simulink model "usrp_1t3r_positioning"  (R2017a)
settings: Solver=VariableStepAuto  StartTime=0.0  StopTime=inf  RelTol=1e-3
undefined symbols (not defined in the file): get
libraries: dspsnks4 x5, commsdrhw_v2 x1, dspxfrm3 x1, dspstat3 x1, dspmtrx3 x1, dspsigops x1
settings Model: SimulationMode=accelerator  Creator=Sky  LastModifiedBy=Sky

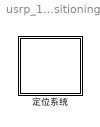
== system usrp_1t3r_positioning ==
  定位系统 : Subsystem  mask{decimInterp=100, fTr=400, nPul=3, tPul=0.1e-3, nCyclePF=5, trEdge=0, antBits=logical([0 0;1 0;0 1])}
      mask prompts: decimInterp "Decimation Factor"; fTr "triger frequency"; nPul "pulse number"; tPul "pulse time"; nCyclePF "cycles per frame (average time)"; trEdge "triger Edge"; antBits "antenna bits"
      mask init:
      | global nRx lF fS lRamp
      | nRx=size(antBits,1);
      | lF=100e6/decimInterp/fTr*nRx*nCyclePF;
      | fS=100e6/decimInterp;
      | lRamp=fS/fTr;%length ramp
      mask TypeOptions decimInterp: USRP/decimInterp
      mask TypeOptions fTr: 定位模块/fTr
      mask TypeOptions nPul: 定位模块/nPul
      mask TypeOptions tPul: 定位模块/tPul
      mask TypeOptions trEdge: 定位模块/trEdge
      mask TypeOptions antBits: 定位模块/antBits
      mask Display: disp('定位系统');

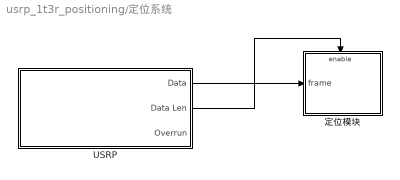
== system usrp_1t3r_positioning/定位系统 ==
  USRP : Subsystem  mask{decimInterp=decimInterp, lF=lF}
      mask prompts: decimInterp "Decimation Factor"; lF "frameLength"
      mask TypeOptions decimInterp: SDRu Receiver/decimInterp
      mask TypeOptions lF: SDRu Receiver/frameLength
      mask Display: disp('USRP');
  定位模块 : Subsystem  mask{fTr=fTr, nPul=nPul, tPul=tPul, trThres=-0.2169682, trEdge=trEdge, antBits=antBits}
      mask prompts: fTr "triger frequency"; nPul "pulse number"; tPul "pulse time"; trThres "triger Threshold"; trEdge "triger Edge"; antBits "antenna bits"
      mask Display: disp('定位模块');
  wires:
  USRP/1(Data) -> 定位模块/1(frame)
  USRP/2(Data Len) -> 定位模块/Enable

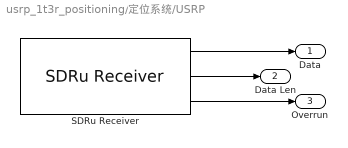
== system usrp_1t3r_positioning/定位系统/USRP ==
  SDRu Receiver : commsdrhw_v2/SDRu Receiver  SourceLibraryInfo="This block requires <a href=\"http://www.mathworks.com/hardware-support/usrp.html\">Communications System Toolbox Support Package for USRP Radio</a>"  rxtx=rx  platform=N200/N210/USRP2  USRP2_IP='192.168.10.6'  USRP_IP_X300='192.168.10.2'  USRP_IP_X310='192.168.10.2'  USRP_serialNumB200=''  USRP_serialNumB210=''  ChannelMapping=1  centerFrequency=0  centerFrequencySrc=Dialog  loOffset=0  loOffsetSrc=Dialog  PPSSource=Internal  clockSource=Internal  masterClkRateB200=32e6  masterClkRateB210=32e6  masterClkRateX300=200e6  masterClkRateX310=200e6  masterClkRateParam=100e6  gain=0  gainSrc=Dialog  decimInterpSrc=Dialog  decimInterp=decimInterp  TransportDataType=int16  USRP2_IP_NUM=[49 57 50 46 49 54 56 46 49 48 46 54]  frameLength=lF  outputDatatype=single  overrunUnderrunPort=on  sampleTime=decimInterp/100e6  HOST_DATA_PORT=0  HOST_CONTROL_PORT=0  USRP2_DATA_PORT=0  USRP2_CONTROL_PORT=0  bufferMode=Continuous streaming  EnableBurstMode=off  NumFramesInBurst=10000  USRP_ID='192.168.10.6'
      settings: SourceProductName=Communications System Toolbox Support Package for USRP(R) Radio  SourceProductBaseCode=USRP
  Data : Outport
  Data Len : Outport  Port=2
  Overrun : Outport  Port=3
  wires:
  SDRu Receiver/2 -> Data Len/1
  SDRu Receiver/3 -> Overrun/1
  SDRu Receiver/1 -> Data/1

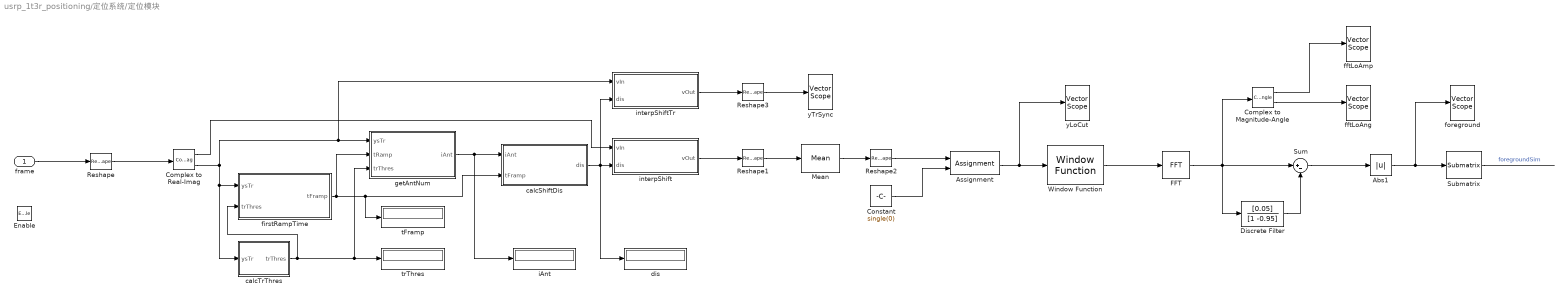
== system usrp_1t3r_positioning/定位系统/定位模块 ==
  frame : Inport
  Enable : EnablePort
  Abs1 : Abs
  Assignment : Assignment  NumberOfDimensions=2  DiagnosticForDimensions=Warning  IndexOptions=Index vector (dialog),Assign all  Indices=[1:ceil(1.5e-5*fS),lRamp-ceil(1.5e-5*fS):lRamp],1  OutputSizes=1,1
  Complex to Magnitude-Angle : ComplexToMagnitudeAngle
  Complex to Real-Imag : ComplexToRealImag
  Constant : Constant  Value=single(0)
  Discrete Filter : DiscreteFilter  Numerator=[0.05]  Denominator=[1 -0.95]
  FFT : dspxfrm3/FFT  FFTImplementation=Auto  CompMethod=Table lookup  TableOpt=NEW  TableOptActive=Speed  BitRevOrder=off  Normalize=off  InheritFFTLength=on  FFTLength=1024*16  WrapInput=on  roundingMode=Floor  overflowMode=off  firstCoeffDataTypeStr=Inherit: Same word length as input  firstCoeffLastDataTypeStr=Inherit: Same word length as input  outputMin=[]  outputMax=[]
  Mean : dspstat3/Mean  run=off  reset_popup=None  InputProcessing=Columns as channels (frame based)  directionMode=Each row  dimension=1  roiEnable=off  roiType=Rectangles  roiPortion=Entire ROI  roiOutput=Individual statistics for each ROI  roiFlag=off  outputDataTypeStr=Inherit: Same as accumulator  outputLastDataTypeStr=Inherit: Same as accumulator  outputMin=[]  outputMax=[]  roundingMode=Floor  overflowMode=off
  Reshape : Reshape  OutputDimensionality=Row vector (2-D)
  Reshape1 : Reshape  OutputDimensionality=Customize  OutputDimensions=[lRamp*nRx,nCyclePF]
  Reshape2 : Reshape  OutputDimensionality=Customize  OutputDimensions=[lRamp,nRx]
  Reshape3 : Reshape  OutputDimensionality=Column vector (2-D)
  Submatrix : dspmtrx3/Submatrix  RowSpan=Range of rows  RowStartMode=First  RowStartIndex=1  RowEndMode=Offset from middle  RowEndIndex=-1  ColSpan=All columns  ColStartMode=First  ColStartIndex=1  ColEndMode=Last  ColEndIndex=1
  Sum : Sum  Inputs=|+-
  Window Function : dspsigops/Window Function  winmode=Apply window to input  wintype=Hanning  sampmode=Continuous  samptime=1  N=64  Rs=50  beta=10  winsamp=Symmetric  UserWindow=hamming  OptParams=off  UserParams={'symmetric'}  dataType=double  isSigned=on  wordLen=16  udDataType=sfix(16)  fracBitsMode=Best precision  numFracBits=15  roundingMode=Floor  overflowMode=off  numSidelobes=4  sidelobeLevel=-30
      settings: SourceProductName=DSP System Toolbox  SourceProductBaseCode=DS
  calcShiftDis : MATLAB Function  TreatAsAtomicUnit=on
  calcTrThres : MATLAB Function  TreatAsAtomicUnit=on
  dis : Display
  fftLoAmp : dspsnks4/Vector Scope  ScopeProperties=on  Domain=Frequency  HorizSpan=1  DisplayProperties=off  AxisGrid=on  Memory=off  FrameNumber=on  AxisLegend=on  AxisZoom=off  OpenScopeAtSimStart=on  OpenScopeImmediately=off  FigPos=get(0,'defaultfigureposition')  AxisProperties=off  XUnits=Hertz  XRange=[0...Fs/2]  InheritXIncr=off  XIncr=1/fS  XLabel=Time  XLimit=Auto  XMin=0  XMax=1  XStart=0  YUnits=Magnitude  YLabel=Amplitude  LineProperties=off  LineDisables=on|on|on  LineColors=[1 0 0]|[0 1 0]|[0 0 1]  XAxisParamsVer=6.9
      settings: SourceProductName=DSP System Toolbox  SourceProductBaseCode=DS  YMin=0  YMax=50
  fftLoAng : dspsnks4/Vector Scope  ScopeProperties=on  Domain=Frequency  HorizSpan=1  DisplayProperties=off  AxisGrid=on  Memory=off  FrameNumber=on  AxisLegend=on  AxisZoom=off  OpenScopeAtSimStart=on  OpenScopeImmediately=off  FigPos=get(0,'defaultfigureposition')  AxisProperties=off  XUnits=Hertz  XRange=[0...Fs/2]  InheritXIncr=off  XIncr=1/fS  XLabel=Time  XLimit=Auto  XMin=0  XMax=1  XStart=0  YUnits=Magnitude  YLabel=Amplitude  LineProperties=off  LineDisables=on|on|on  LineColors=[1 0 0]|[0 1 0]|[0 0 1]  XAxisParamsVer=6.9
      settings: SourceProductName=DSP System Toolbox  SourceProductBaseCode=DS  YMin=-4  YMax=4
  firstRampTime : MATLAB Function  TreatAsAtomicUnit=on
  foreground : dspsnks4/Vector Scope  ScopeProperties=on  Domain=Frequency  HorizSpan=1  DisplayProperties=off  AxisGrid=on  Memory=off  FrameNumber=on  AxisLegend=on  AxisZoom=off  OpenScopeAtSimStart=on  OpenScopeImmediately=off  FigPos=get(0,'defaultfigureposition')  AxisProperties=off  XUnits=Hertz  XRange=[0...Fs/2]  InheritXIncr=off  XIncr=1/fS  XLabel=Time  XLimit=Auto  XMin=0  XMax=1  XStart=0  YUnits=Magnitude  YLabel=Amplitude  LineProperties=off  LineDisables=on|on|on  LineColors=[1 0 0]|[0 1 0]|[0 0 1]  XAxisParamsVer=6.9
      settings: SourceProductName=DSP System Toolbox  SourceProductBaseCode=DS  YMin=0  YMax=0.2
  getAntNum : MATLAB Function  TreatAsAtomicUnit=on
  iAnt : Display
  interpShift : MATLAB Function  TreatAsAtomicUnit=on
  interpShiftTr : MATLAB Function  TreatAsAtomicUnit=on
  tFramp : Display
  trThres : Display
  yLoCut : dspsnks4/Vector Scope  ScopeProperties=on  Domain=Time  HorizSpan=1  DisplayProperties=off  AxisGrid=on  Memory=off  FrameNumber=on  AxisLegend=off  AxisZoom=off  OpenScopeAtSimStart=on  OpenScopeImmediately=off  FigPos=get(0,'defaultfigureposition')  AxisProperties=off  XUnits=Hertz  XRange=[0...Fs/2]  InheritXIncr=on  XIncr=1  XLabel=Time  XLimit=Auto  XMin=0  XMax=1  XStart=0  YUnits=dB  YLabel=Amplitude  LineProperties=off  LineColors=[1 0 0]|[0 1 0]|[0 0 1]  XAxisParamsVer=6.9
      settings: SourceProductName=DSP System Toolbox  SourceProductBaseCode=DS  YMin=-0.5  YMax=0.5
  yTrSync : dspsnks4/Vector Scope  ScopeProperties=on  Domain=Time  HorizSpan=1  DisplayProperties=off  AxisGrid=on  Memory=off  FrameNumber=on  AxisLegend=off  AxisZoom=off  OpenScopeAtSimStart=on  OpenScopeImmediately=off  FigPos=get(0,'defaultfigureposition')  AxisProperties=off  XUnits=Hertz  XRange=[0...Fs/2]  InheritXIncr=on  XIncr=1  XLabel=Time  XLimit=Auto  XMin=0  XMax=1  XStart=0  YUnits=dB  YLabel=Amplitude  LineProperties=off  LineColors=[1 0 0]|[0 1 0]|[0 0 1]  XAxisParamsVer=6.9
      settings: SourceProductName=DSP System Toolbox  SourceProductBaseCode=DS  YMin=-0.6  YMax=0.2
  wires:
  firstRampTime/1(tFramp) -> tFramp/1, calcShiftDis/2(tFramp), getAntNum/2(tRamp)
  frame/1 -> Reshape/1
  Reshape/1 -> Complex to Real-Imag/1
  getAntNum/1(iAnt) -> iAnt/1, calcShiftDis/1(iAnt)
  Complex to Real-Imag/2 -> calcTrThres/1(ysTr), firstRampTime/1(ysTr), interpShiftTr/1(vIn), getAntNum/1(ysTr)
  calcShiftDis/1(dis) -> dis/1, interpShift/2(dis), interpShiftTr/2(dis)
  interpShift/1(vOut) -> Reshape1/1
  Complex to Real-Imag/1 -> interpShift/1(vIn)
  calcTrThres/1(trThres) -> trThres/1, getAntNum/3(trThres), firstRampTime/2(trThres)
  Reshape1/1 -> Mean/1
  Mean/1 -> Reshape2/1
  Discrete Filter/1 -> Sum/2
  FFT/1 -> Complex to Magnitude-Angle/1, Discrete Filter/1, Sum/1
  Sum/1 -> Abs1/1
  Abs1/1 -> Submatrix/1, foreground/1
  Complex to Magnitude-Angle/2 -> fftLoAng/1
  Reshape2/1 -> Assignment/1
  Constant/1 -> Assignment/2
  Submatrix/1 -> ?  "foregroundSim"
  Assignment/1 -> yLoCut/1, Window Function/1
  Complex to Magnitude-Angle/1 -> fftLoAmp/1
  interpShiftTr/1(vOut) -> Reshape3/1
  Reshape3/1 -> yTrSync/1
  Window Function/1 -> FFT/1

== matlab function usrp_1t3r_positioning/定位系统/定位模块/getAntNum ==
  data: ysTr input; tRamp input; iAnt output; fS parameter; tPul parameter; antBits parameter; trThres input
%% 判断触发时间对应同步信号的天线编号
% iAnt: 天线编号
% ysTr: 一帧triger信号
% tRamp: 斜坡开始时间，以第一个采样点为参考时间0
% fS: 采样率
% tPul: 脉冲/比特宽度
% trThres: 触发电平
% antBits: 天线编号
function iAnt=getAntNum(ysTr, tRamp, fS, tPul, antBits, trThres)
if isnan(tRamp)
    iAnt=nan;
    return
end
%% 准备参数
lPul=fS*tPul;%length pulse

%% 抽取天线编号的比特电平
iBit1=ceil((tRamp+1.5*tPul)*fS)+1;
isBits=linspace(iBit1,iBit1+lPul*(size(antBits,2)-1),size(antBits,2));

ysBits=ysTr(isBits);
isAnt=find(all(~xor(antBits,repmat((ysBits>trThres),size(antBits,1),1)),2),1);
if isempty(isAnt)
    iAnt=nan;
    return
end
iAnt=isAnt(1);%为simulink推理iAnt大小提供帮助

end

== matlab function usrp_1t3r_positioning/定位系统/定位模块/firstRampTime ==
  data: ysTr input; tFramp output; fS parameter; fTr parameter; tPul parameter; nPul parameter; trEdge parameter; trThres input
%% 同步斜坡信号起始时间函数，返回所有斜坡信号起始时间点
% tFramp: 第一个斜坡开始时间，精确到采样时间之下，以第一个采样点为参考时间0
% ysTr: 一帧triger信号
% fS: 采样率
% fTr: 触发信号频率
% tPul: 脉冲/比特宽度
% nPul: 脉冲/比特总数
% trEdge: 触发沿：1上升沿 0下降沿
% trThres: 触发电平
function tFramp=firstRampTime(ysTr, fS, fTr, tPul, nPul, trEdge, trThres)
%% 准备参数
lRamp=fS/fTr;%length ramp
lPul=fS*tPul;%length pulse

if(mod(size(ysTr,2),lRamp)~=0)
    error('The length of frame is not integer multiple of the length of ramp .');
end

%% 分析第一个完整斜坡同步信号
%第一个完整斜坡同步信号触发沿位于1:lRamp,为了容错，扩大范围到1:lRamp+lPul*nPul
isFramp=1:lRamp+lPul*nPul;%indexs first ramp
ysTrFf=ysTr(isFramp);%ys triger first ramp
isTrF=[];
if trEdge==0
    isTrF=find(ysTrFf(2:end)<trThres & ysTrFf(1:end-1)>=trThres)+1;%index triger first
else
    isTrF=find(ysTrFf(2:end)>trThres & ysTrFf(1:end-1)<=trThres)+1;
end
if isempty(isTrF)
    tFramp=single(nan);
    return
else
    iTrF=isTrF(find([true diff(isTrF)>lPul*nPul],1,'last'));%要求脉冲和比特总时长小于斜坡周期的一半,选取最后一个触发信号
end

% 在调试错误触发时启用
% if ysTr(iTrF+150)>trThres && ysTr(iTrF+250)>trThres
%     tFramp=single(nan);
%     return
% end

%% 线性插值分析上升沿的精确时间
tFramp=interp1([ysTr(iTrF-1),ysTr(iTrF)],([iTrF-1,iTrF]-1)/fS,trThres);
end

== matlab function usrp_1t3r_positioning/定位系统/定位模块/interpShiftTr ==
  data: vIn input; vOut output; dis input
%% 循环移位，通过线性插值实现小数位数的移位
% vOut: 输出向量
% vIn: 输入向量
% dis: 向右移位距离
function vOut=interpShift(vIn, dis)
    if isnan(dis)
        vOut=vIn;
        return
    end
    isZeroBased=0:length(vIn)-1;
    if dis>=0
        iShift=floor(dis);
        iAdd=dis-iShift;
    else
        iShift=ceil(dis);
        iAdd=iShift-dis;
    end
    
    isShifted=circshift(isZeroBased,iShift);
    iInterp=isShifted+iAdd;
    vOut=interp1(isZeroBased,vIn,iInterp,'linear','extrap');
end

== matlab function usrp_1t3r_positioning/定位系统/定位模块/calcShiftDis ==
  data: iAnt input; dis output; tFramp input; lRamp parameter; fS parameter; nRx parameter
%% 通过天线序号、时间偏移计算循环移位位移量
% dis: 位移量
% iAnt: 天线序号，从1开始
% tFramp: 第一个触发信号时间
% fS: 采样率
% nRx: 天线数量
function dis=calcShiftDis(iAnt,tFramp,lRamp,fS,nRx)
    dis=-((nRx+1-iAnt)*lRamp+(tFramp*fS));
end

== matlab function usrp_1t3r_positioning/定位系统/定位模块/interpShift ==
  data: vIn input; vOut output; dis input
%% 循环移位，通过线性插值实现小数位数的移位
% vOut: 输出向量
% vIn: 输入向量
% dis: 向右移位距离
function vOut=interpShift(vIn, dis)
    if isnan(dis)
        vOut=vIn;
        return
    end
    isZeroBased=0:length(vIn)-1;
    if dis>=0
        iShift=floor(dis);
        iAdd=dis-iShift;
    else
        iShift=ceil(dis);
        iAdd=iShift-dis;
    end
    
    isShifted=circshift(isZeroBased,iShift);
    iInterp=isShifted+iAdd;
    vOut=interp1(isZeroBased,vIn,iInterp,'linear','extrap');
end

== matlab function usrp_1t3r_positioning/定位系统/定位模块/calcTrThres ==
  data: ysTr input; trThres output
%% 计算触发电平
function trThres = calcTrThres(ysTr)
trThres=(max(ysTr)+min(ysTr))/2;%triger threshold
% trThres=(mean(ysTr(ysTr>trThres))+mean(ysTr(ysTr<trThres)))/2;
end
